simulink model "inverter_network"  (R2023a)
settings: Solver=ode4  StartTime=0.0  StopTime=0.8  FixedStep=1e-6  RelTol=1e-3
values from neighbouring files (symbols this model uses):
  C_gv = 1.5e-3    (= 0.0015)    [init.m]
  Cf = 2e-5    (= 2e-05)    [init.m]
  Cf_r = 1    [init.m]
  frequency = 50    [init.m]
  kpgi = 15    [init.m]
  kpi = 8    [init.m]
  kpv = 0.1    [init.m]
  krgi = 600    [init.m]
  krv = 100    [init.m]
  L_fv = 1.5e-3    (= 0.0015)    [init.m]
  L_line = 0.003*rbase/omega    (= 0.000152788745368)    [init.m]
  Lf = 4e-3    (= 0.004)    [init.m]
  Lf_r = 0.3    [init.m]
  Lg = 0.24e-3    (= 0.00024)    [init.m]
  omega = 2*pi*frequency    (= 314.159265359)    [init.m]
  R_line = 0.013*rbase    (= 0.208)    [init.m]
  vc_l = 0.03*rbase    (= 0.48)    [init.m]
  vdc = 400*1.88    (= 752)    [init.m]
  vref_rms = 300*(0.707*sqrt(3))    [init.m]
libraries: spsThreePhaseVIMeasurementLib x14, spsHalfBridgeConverterLib x9, spsThreePhaseSeriesRLCBranchLib x7, spsPower3phInstantaneousLib x6, spsThreePhaseParallelRLCBranchLib x5, spsabctoAlphaBetaZeroLib x5, spsGroundLib x4, spsAlphaBetaZerotoabcLib x3, spsDCVoltageSourceLib x3, eePwmGeneratorTwoLevel x3, spsPLL3phLib x2, spsdq0toAlphaBetaZeroLib x2
(part 2 of 2)

== system inverter_network/Current Controlled VSC2/Subsystem7 ==
  Three-Phase V-I Measurement2 : spsThreePhaseVIMeasurementLib/Three-Phase V-I Measurement  VoltageMeasurement=phase-to-ground  SetLabelV=off  LabelV=Vabc  Vpu=off  VpuLL=off  CurrentMeasurement=yes  SetLabelI=off  LabelI=Iabc  Ipu=off  Pbase=100e6  Vbase=500e3  OutputType=Complex  PhasorSimulation=off  PSBequivalent=0
  A : PMIOPort  Side=Left
  B : PMIOPort  Port=2  Side=Left
  C : PMIOPort  Port=3  Side=Left
  a : PMIOPort  Port=4  Side=Right
  b : PMIOPort  Port=5  Side=Right
  c : PMIOPort  Port=6  Side=Right
  Iabc : Outport
  wires:
  Three-Phase V-I Measurement2/2 -> Iabc/1
  connections:
  Three-Phase V-I Measurement2/LConn1 -- A/RConn1
  Three-Phase V-I Measurement2/RConn3 -- c/RConn1
  Three-Phase V-I Measurement2/RConn1 -- a/RConn1
  Three-Phase V-I Measurement2/LConn2 -- B/RConn1
  Three-Phase V-I Measurement2/RConn2 -- b/RConn1
  Three-Phase V-I Measurement2/LConn3 -- C/RConn1

== system inverter_network/Current Controlled VSC2/Subsystem8 ==
  Three-Phase V-I Measurement3 : spsThreePhaseVIMeasurementLib/Three-Phase V-I Measurement  VoltageMeasurement=phase-to-ground  SetLabelV=off  LabelV=Vabc  Vpu=off  VpuLL=off  CurrentMeasurement=yes  SetLabelI=off  LabelI=Iabc  Ipu=off  Pbase=100e6  Vbase=500e3  OutputType=Complex  PhasorSimulation=off  PSBequivalent=0
  A : PMIOPort  Side=Left
  B : PMIOPort  Port=2  Side=Left
  C : PMIOPort  Port=3  Side=Left
  Vabc : Outport
  wires:
  Three-Phase V-I Measurement3/1 -> Vabc/1
  connections:
  Three-Phase V-I Measurement3/LConn1 -- A/RConn1
  Three-Phase V-I Measurement3/LConn2 -- B/RConn1
  Three-Phase V-I Measurement3/LConn3 -- C/RConn1

== system inverter_network/Current Controlled VSC2/Subsystem9 ==
  Three-Phase V-I Measurement : spsThreePhaseVIMeasurementLib/Three-Phase V-I Measurement  VoltageMeasurement=phase-to-ground  SetLabelV=off  LabelV=Vabc  Vpu=off  VpuLL=off  CurrentMeasurement=yes  SetLabelI=off  LabelI=Iabc  Ipu=off  Pbase=100e6  Vbase=500e3  OutputType=Complex  PhasorSimulation=off  PSBequivalent=0
  A : PMIOPort  Side=Left
  B : PMIOPort  Port=2  Side=Left
  C : PMIOPort  Port=3  Side=Left
  a : PMIOPort  Port=4  Side=Right
  b : PMIOPort  Port=5  Side=Right
  c : PMIOPort  Port=6  Side=Right
  Vabc : Outport
  Iabc : Outport  Port=2
  wires:
  Three-Phase V-I Measurement/2 -> Iabc/1
  Three-Phase V-I Measurement/1 -> Vabc/1
  connections:
  Three-Phase V-I Measurement/RConn1 -- a/RConn1
  Three-Phase V-I Measurement/LConn2 -- B/RConn1
  Three-Phase V-I Measurement/RConn3 -- c/RConn1
  Three-Phase V-I Measurement/LConn1 -- A/RConn1
  Three-Phase V-I Measurement/LConn3 -- C/RConn1
  Three-Phase V-I Measurement/RConn2 -- b/RConn1

== system inverter_network/Current Controlled VSC2/dq0 to Alpha Beta1 ==
  dq0 : Inport
  wt : Inport  Port=2
  dq0 to Alpha-Beta-Zero : spsdq0toAlphaBetaZeroLib/dq0 to Alpha-Beta-Zero  Alignment=90 degrees behind phase A axis
  al_be_0 : Outport
  wires:
  dq0 to Alpha-Beta-Zero/1 -> al_be_0/1
  wt/1 -> dq0 to Alpha-Beta-Zero/2
  dq0/1 -> dq0 to Alpha-Beta-Zero/1

== system inverter_network/Subsystem/Subsystem10 ==
  Three-Phase V-I Measurement : spsThreePhaseVIMeasurementLib/Three-Phase V-I Measurement  VoltageMeasurement=phase-to-ground  SetLabelV=off  LabelV=Vabc  Vpu=off  VpuLL=off  CurrentMeasurement=yes  SetLabelI=off  LabelI=Iabc  Ipu=off  Pbase=100e6  Vbase=500e3  OutputType=Complex  PhasorSimulation=off  PSBequivalent=0
  A : PMIOPort  Side=Left
  B : PMIOPort  Port=2  Side=Left
  C : PMIOPort  Port=3  Side=Left
  a : PMIOPort  Port=4  Side=Right
  b : PMIOPort  Port=5  Side=Right
  c : PMIOPort  Port=6  Side=Right
  Vabc : Outport
  Iabc : Outport  Port=2
  wires:
  Three-Phase V-I Measurement/2 -> Iabc/1
  Three-Phase V-I Measurement/1 -> Vabc/1
  connections:
  Three-Phase V-I Measurement/RConn1 -- a/RConn1
  Three-Phase V-I Measurement/LConn2 -- B/RConn1
  Three-Phase V-I Measurement/RConn3 -- c/RConn1
  Three-Phase V-I Measurement/LConn1 -- A/RConn1
  Three-Phase V-I Measurement/LConn3 -- C/RConn1
  Three-Phase V-I Measurement/RConn2 -- b/RConn1

== system inverter_network/Subsystem2/Subsystem10 ==
  Three-Phase V-I Measurement : spsThreePhaseVIMeasurementLib/Three-Phase V-I Measurement  VoltageMeasurement=phase-to-ground  SetLabelV=off  LabelV=Vabc  Vpu=off  VpuLL=off  CurrentMeasurement=yes  SetLabelI=off  LabelI=Iabc  Ipu=off  Pbase=100e6  Vbase=500e3  OutputType=Complex  PhasorSimulation=off  PSBequivalent=0
  A : PMIOPort  Side=Left
  B : PMIOPort  Port=2  Side=Left
  C : PMIOPort  Port=3  Side=Left
  a : PMIOPort  Port=4  Side=Right
  b : PMIOPort  Port=5  Side=Right
  c : PMIOPort  Port=6  Side=Right
  Vabc : Outport
  Iabc : Outport  Port=2
  wires:
  Three-Phase V-I Measurement/2 -> Iabc/1
  Three-Phase V-I Measurement/1 -> Vabc/1
  connections:
  Three-Phase V-I Measurement/RConn1 -- a/RConn1
  Three-Phase V-I Measurement/LConn2 -- B/RConn1
  Three-Phase V-I Measurement/RConn3 -- c/RConn1
  Three-Phase V-I Measurement/LConn1 -- A/RConn1
  Three-Phase V-I Measurement/LConn3 -- C/RConn1
  Three-Phase V-I Measurement/RConn2 -- b/RConn1

== system inverter_network/Subsystem3/Subsystem10 ==
  Three-Phase V-I Measurement : spsThreePhaseVIMeasurementLib/Three-Phase V-I Measurement  VoltageMeasurement=phase-to-ground  SetLabelV=off  LabelV=Vabc  Vpu=off  VpuLL=off  CurrentMeasurement=yes  SetLabelI=off  LabelI=Iabc  Ipu=off  Pbase=100e6  Vbase=500e3  OutputType=Complex  PhasorSimulation=off  PSBequivalent=0
  A : PMIOPort  Side=Left
  B : PMIOPort  Port=2  Side=Left
  C : PMIOPort  Port=3  Side=Left
  a : PMIOPort  Port=4  Side=Right
  b : PMIOPort  Port=5  Side=Right
  c : PMIOPort  Port=6  Side=Right
  Vabc : Outport
  Iabc : Outport  Port=2
  wires:
  Three-Phase V-I Measurement/2 -> Iabc/1
  Three-Phase V-I Measurement/1 -> Vabc/1
  connections:
  Three-Phase V-I Measurement/RConn1 -- a/RConn1
  Three-Phase V-I Measurement/LConn2 -- B/RConn1
  Three-Phase V-I Measurement/RConn3 -- c/RConn1
  Three-Phase V-I Measurement/LConn1 -- A/RConn1
  Three-Phase V-I Measurement/LConn3 -- C/RConn1
  Three-Phase V-I Measurement/RConn2 -- b/RConn1

== system inverter_network/Subsystem4/Subsystem10 ==
  Three-Phase V-I Measurement : spsThreePhaseVIMeasurementLib/Three-Phase V-I Measurement  VoltageMeasurement=phase-to-ground  SetLabelV=off  LabelV=Vabc  Vpu=off  VpuLL=off  CurrentMeasurement=yes  SetLabelI=off  LabelI=Iabc  Ipu=off  Pbase=100e6  Vbase=500e3  OutputType=Complex  PhasorSimulation=off  PSBequivalent=0
  A : PMIOPort  Side=Left
  B : PMIOPort  Port=2  Side=Left
  C : PMIOPort  Port=3  Side=Left
  a : PMIOPort  Port=4  Side=Right
  b : PMIOPort  Port=5  Side=Right
  c : PMIOPort  Port=6  Side=Right
  Vabc : Outport
  Iabc : Outport  Port=2
  wires:
  Three-Phase V-I Measurement/2 -> Iabc/1
  Three-Phase V-I Measurement/1 -> Vabc/1
  connections:
  Three-Phase V-I Measurement/RConn1 -- a/RConn1
  Three-Phase V-I Measurement/LConn2 -- B/RConn1
  Three-Phase V-I Measurement/RConn3 -- c/RConn1
  Three-Phase V-I Measurement/LConn1 -- A/RConn1
  Three-Phase V-I Measurement/LConn3 -- C/RConn1
  Three-Phase V-I Measurement/RConn2 -- b/RConn1

== system inverter_network/Subsystem5/Subsystem10 ==
  Three-Phase V-I Measurement : spsThreePhaseVIMeasurementLib/Three-Phase V-I Measurement  VoltageMeasurement=phase-to-ground  SetLabelV=off  LabelV=Vabc  Vpu=off  VpuLL=off  CurrentMeasurement=yes  SetLabelI=off  LabelI=Iabc  Ipu=off  Pbase=100e6  Vbase=500e3  OutputType=Complex  PhasorSimulation=off  PSBequivalent=0
  A : PMIOPort  Side=Left
  B : PMIOPort  Port=2  Side=Left
  C : PMIOPort  Port=3  Side=Left
  a : PMIOPort  Port=4  Side=Right
  b : PMIOPort  Port=5  Side=Right
  c : PMIOPort  Port=6  Side=Right
  Vabc : Outport
  Iabc : Outport  Port=2
  wires:
  Three-Phase V-I Measurement/2 -> Iabc/1
  Three-Phase V-I Measurement/1 -> Vabc/1
  connections:
  Three-Phase V-I Measurement/RConn1 -- a/RConn1
  Three-Phase V-I Measurement/LConn2 -- B/RConn1
  Three-Phase V-I Measurement/RConn3 -- c/RConn1
  Three-Phase V-I Measurement/LConn1 -- A/RConn1
  Three-Phase V-I Measurement/LConn3 -- C/RConn1
  Three-Phase V-I Measurement/RConn2 -- b/RConn1

== system inverter_network/Voltage Controlled VSC/PR Control1 ==
  In1 : Inport
  Constant2 : Constant  Value=0
  Demux3 : Demux  Outputs=3
  Mux4 : Mux  Inputs=3
  Terminator : Terminator
  Transfer Fcn : TransferFcn  Numerator=[kpv krv kpv*(omega^2)]  Denominator=[1 0 omega^2]
  Transfer Fcn1 : TransferFcn  Numerator=[kpv krv kpv*(omega^2)]  Denominator=[1 0 omega^2]
  Out1 : Outport
  wires:
  Transfer Fcn/1 -> Mux4/1
  Mux4/1 -> Out1/1
  Demux3/1 -> Transfer Fcn/1
  Demux3/2 -> Transfer Fcn1/1
  Constant2/1 -> Mux4/3
  Transfer Fcn1/1 -> Mux4/2
  In1/1 -> Demux3/1
  Demux3/3 -> Terminator/1

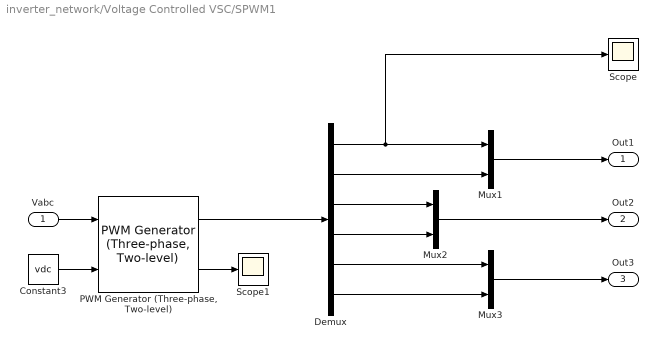
== system inverter_network/Voltage Controlled VSC/SPWM1 ==
  Vabc : Inport
  Constant3 : Constant  Value=vdc
  Demux : Demux  Outputs=6
  Mux1 : Mux  Inputs=2
  Mux2 : Mux  Inputs=2
  Mux3 : Mux  Inputs=2
  "PWM Generator (Three-phase, Two-level)" : eePwmGeneratorTwoLevel/PWM Generator (Three-phase, Two-level)  PWMMode=Continuous PWM (CPWM)  CPWMMode=SPWM: sinusoidal PWM  DPWMMode=60 DPWM: 60 degree discontinuous PWM  fsw=fsw  Ts=1/(100*10000)
      settings: LibrarySourceBlock=|
      | ee_sl_lib/Pulse Width
      | Modulation/PWM Generator
      | (Three-phase, Two-level)
  Scope : Scope
  Scope1 : Scope
  Out1 : Outport
  Out2 : Outport  Port=2
  Out3 : Outport  Port=3
  wires:
  "PWM Generator (Three-phase, Two-level)"/2 -> Scope1/1
  Demux/2 -> Mux1/2
  Vabc/1 -> "PWM Generator (Three-phase, Two-level)"/1
  Demux/6 -> Mux3/2
  Demux/1 -> Scope/1, Mux1/1
  Constant3/1 -> "PWM Generator (Three-phase, Two-level)"/2
  Mux2/1 -> Out2/1
  Demux/4 -> Mux2/2
  "PWM Generator (Three-phase, Two-level)"/1 -> Demux/1
  Demux/3 -> Mux2/1
  Demux/5 -> Mux3/1
  Mux1/1 -> Out1/1
  Mux3/1 -> Out3/1

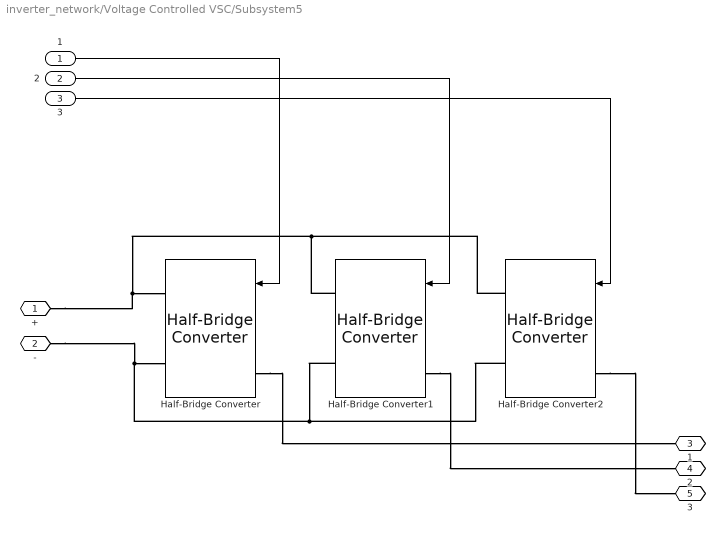
== system inverter_network/Voltage Controlled VSC/Subsystem5 ==
  " 1 " : Inport
  "  2" : Inport  Port=2
  "  3" : Inport  Port=3
  Half-Bridge Converter : spsHalfBridgeConverterLib/Half-Bridge Converter  ModelType=Switching devices  Ron=1e-3  Rs=1e6  Cs=inf  Vforward=[0,0]  Ron_Diode=1e-3  Rs_Diode=1e6  Cs_Diode=inf  Vf_Diode=1e-3  Rs_CurrentSource=inf  Ron_ACsource=1e-3
      settings: LibrarySourceBlock=sps_lib/Power Electronics/Half-Bridge Converter
  Half-Bridge Converter1 : spsHalfBridgeConverterLib/Half-Bridge Converter  ModelType=Switching devices  Ron=1e-3  Rs=1e6  Cs=inf  Vforward=[0,0]  Ron_Diode=1e-3  Rs_Diode=1e6  Cs_Diode=inf  Vf_Diode=1e-3  Rs_CurrentSource=inf  Ron_ACsource=1e-3
      settings: LibrarySourceBlock=sps_lib/Power Electronics/Half-Bridge Converter
  Half-Bridge Converter2 : spsHalfBridgeConverterLib/Half-Bridge Converter  ModelType=Switching devices  Ron=1e-3  Rs=1e6  Cs=inf  Vforward=[0,0]  Ron_Diode=1e-3  Rs_Diode=1e6  Cs_Diode=inf  Vf_Diode=1e-3  Rs_CurrentSource=inf  Ron_ACsource=1e-3
      settings: LibrarySourceBlock=sps_lib/Power Electronics/Half-Bridge Converter
  + : PMIOPort  Side=Left
  - : PMIOPort  Port=2  Side=Left
  1 : PMIOPort  Port=3  Side=Right
  2 : PMIOPort  Port=4  Side=Right
  3 : PMIOPort  Port=5  Side=Right
  wires:
  "  2"/1 -> Half-Bridge Converter1/1
  "  3"/1 -> Half-Bridge Converter2/1
  " 1 "/1 -> Half-Bridge Converter/1
  connections:
  Half-Bridge Converter/LConn1 -- 1/RConn1
  Half-Bridge Converter1/RConn1 -- Half-Bridge Converter2/RConn1 -- +/RConn1 -- Half-Bridge Converter/RConn1
  Half-Bridge Converter2/RConn2 -- Half-Bridge Converter1/RConn2 -- -/RConn1 -- Half-Bridge Converter/RConn2
  Half-Bridge Converter2/LConn1 -- 3/RConn1
  Half-Bridge Converter1/LConn1 -- 2/RConn1

== system inverter_network/Voltage Controlled VSC/Vref ==
  Ground4 : spsGroundLib/Ground  LConnTagsString=a
  Three-Phase Programmable Voltage Source1 : spsThreePhaseProgrammableVoltageSourceLib/Three-Phase Programmable Voltage Source  PositiveSequence="[vref_rms  0 frequency]"  VariationEntity=None  VariationType=Table of time-amplitude pairs  VariationTypeAlt=Step  VariationStep=0.5  VariationRate=10  VariationMagnitude=0.3  VariationFrequency=2  VariationTiming=[1 2]  VariationPhaseA=off  Amplitudes=[1 0.8 1.2 1.0]  TimeValues=[0 0.1 0.15 0.2]  HarmonicGeneration=off  HarmonicA=[3 0.2 -25 0]  HarmonicB=[2 0.15 35 2]  Timing="[0.05  3]"  BusType=swing  Pref=0  Qref=0  Qmin=-inf  Qmax=inf
  Three-Phase V-I Measurement4 : spsThreePhaseVIMeasurementLib/Three-Phase V-I Measurement  VoltageMeasurement=phase-to-ground  SetLabelV=off  LabelV=Vabc  Vpu=off  VpuLL=off  CurrentMeasurement=yes  SetLabelI=off  LabelI=Iabc  Ipu=off  Pbase=100e6  Vbase=500e3  OutputType=Complex  PhasorSimulation=off  PSBequivalent=0
  Vabc : Outport
  wires:
  Three-Phase V-I Measurement4/1 -> Vabc/1
  connections:
  Three-Phase Programmable Voltage Source1/RConn2 -- Three-Phase V-I Measurement4/LConn2
  Three-Phase Programmable Voltage Source1/RConn3 -- Three-Phase V-I Measurement4/LConn3
  Three-Phase Programmable Voltage Source1/RConn1 -- Three-Phase V-I Measurement4/LConn1
  Ground4/LConn1 -- Three-Phase Programmable Voltage Source1/LConn1

== system inverter_network/Current Controlled VSC1/PR Control2/Subsystem ==
  In1 : Inport
  Gain : Gain  Gain=kpgi
  Sum : Sum  Inputs=|++
  Transfer Fcn : TransferFcn  Numerator=[krgi 0]  Denominator=[1 1.2566e-05 omega^2]
  Out1 : Outport
  wires:
  Sum/1 -> Out1/1
  In1/1 -> Transfer Fcn/1, Gain/1
  Transfer Fcn/1 -> Sum/1
  Gain/1 -> Sum/2

== system inverter_network/Current Controlled VSC1/PR Control2/Subsystem1 ==
  In1 : Inport
  Gain : Gain  Gain=kpgi
  Sum : Sum  Inputs=|++
  Transfer Fcn : TransferFcn  Numerator=[krgi 0]  Denominator=[1 1.2566e-05 omega^2]
  Out1 : Outport
  wires:
  Sum/1 -> Out1/1
  In1/1 -> Transfer Fcn/1, Gain/1
  Transfer Fcn/1 -> Sum/1
  Gain/1 -> Sum/2

== system inverter_network/Current Controlled VSC2/PR Control2/Subsystem ==
  In1 : Inport
  Gain : Gain  Gain=kpgi
  Sum : Sum  Inputs=|++
  Transfer Fcn : TransferFcn  Numerator=[krgi 0]  Denominator=[1 1.2566e-05 omega^2]
  Out1 : Outport
  wires:
  Sum/1 -> Out1/1
  In1/1 -> Transfer Fcn/1, Gain/1
  Transfer Fcn/1 -> Sum/1
  Gain/1 -> Sum/2

== system inverter_network/Current Controlled VSC2/PR Control2/Subsystem1 ==
  In1 : Inport
  Gain : Gain  Gain=kpgi
  Sum : Sum  Inputs=|++
  Transfer Fcn : TransferFcn  Numerator=[krgi 0]  Denominator=[1 1.2566e-05 omega^2]
  Out1 : Outport
  wires:
  Sum/1 -> Out1/1
  In1/1 -> Transfer Fcn/1, Gain/1
  Transfer Fcn/1 -> Sum/1
  Gain/1 -> Sum/2
